simulink model "OneLeg_VR_TouchInput"  (Simulink 7.3)
settings: Solver=ode15s  StartTime=0.0  StopTime=inf  RelTol=1e-3
PreLoadFcn:
  | init_hopper
PostLoadFcn:
  | vrmfunc('FnOpen', [bdroot, '/Data Display and Analysis/VR Sink']);
undefined symbols (not defined in the file or in its folder): body, ctrl, ground, leg, sfuntraj, sigbuilder_block, Traj
libraries: mblibv1 x27, dspmtrx3 x8, simulink x4, vrlib x1
(part 2 of 2)

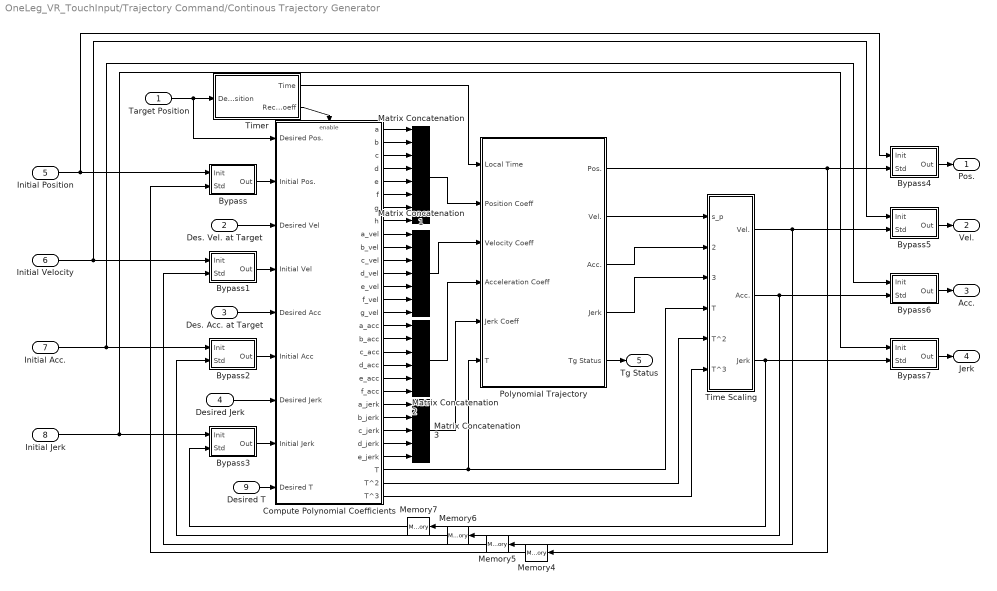
== system OneLeg_VR_TouchInput/Trajectory Command/Continous Trajectory Generator ==
  Target Position : Inport  OutDataType=sfix(16)  OutScaling=2^0
  Des. Vel. at Target : Inport  Port=2  OutDataType=sfix(16)  OutScaling=2^0
  Des. Acc. at Target : Inport  Port=3  OutDataType=sfix(16)  OutScaling=2^0
  Desired Jerk : Inport  Port=4  OutDataType=sfix(16)  OutScaling=2^0
  Initial Position : Inport  Port=5  OutDataType=sfix(16)  OutScaling=2^0
  Initial Velocity : Inport  Port=6  OutDataType=sfix(16)  OutScaling=2^0
  Initial Acc. : Inport  Port=7  OutDataType=sfix(16)  OutScaling=2^0
  Initial Jerk : Inport  Port=8  OutDataType=sfix(16)  OutScaling=2^0
  Desired T : Inport  Port=9  OutDataType=sfix(16)  OutScaling=2^0
  Bypass : Subsystem
  Bypass1 : Subsystem
  Bypass2 : Subsystem
  Bypass3 : Subsystem
  Bypass4 : Subsystem
  Bypass5 : Subsystem
  Bypass6 : Subsystem
  Bypass7 : Subsystem
  Compute Polynomial Coefficients : Subsystem  TreatAsAtomicUnit=on
  Matrix Concatenation : Concatenate  NumInputs=8  Mode=Multidimensional array
  Matrix Concatenation1 : Concatenate  NumInputs=7  Mode=Multidimensional array
  Matrix Concatenation2 : Concatenate  NumInputs=6  Mode=Multidimensional array
  Matrix Concatenation3 : Concatenate  NumInputs=5  Mode=Multidimensional array
  Memory{4..7} (4 alike) : Memory  InheritSampleTime=on
  Polynomial Trajectory : Subsystem  TreatAsAtomicUnit=on
  Time Scaling : Subsystem
  Timer : Subsystem
  Pos. : Outport
  Vel. : Outport  Port=2
  Acc. : Outport  Port=3
  Jerk : Outport  Port=4
  Tg Status : Outport  Port=5
  wires:
  Bypass7/1(Out) -> Jerk/1
  Bypass6/1(Out) -> Acc./1
  Bypass5/1(Out) -> Vel./1
  Bypass4/1(Out) -> Pos./1
  Memory7/1 -> Bypass3/2(Std)
  Memory6/1 -> Bypass2/2(Std)
  Memory5/1 -> Bypass1/2(Std)
  Memory4/1 -> Bypass/2(Std)
  Initial Jerk/1 -> Bypass7/1(Init), Bypass3/1(Init)
  Initial Acc./1 -> Bypass6/1(Init), Bypass2/1(Init)
  Initial Velocity/1 -> Bypass5/1(Init), Bypass1/1(Init)
  Bypass/1(Out) -> Compute Polynomial Coefficients/2(Initial Pos.)
  Initial Position/1 -> Bypass4/1(Init), Bypass/1(Init)
  Compute Polynomial Coefficients/29(T^3) -> Time Scaling/6(T^3)
  Compute Polynomial Coefficients/28(T^2) -> Time Scaling/5(T^2)
  Time Scaling/3(Jerk) -> Bypass7/2(Std), Memory7/1
  Polynomial Trajectory/4(Jerk) -> Time Scaling/3(s_ppp)
  Matrix Concatenation3/1 -> Polynomial Trajectory/5(Jerk Coeff)
  Matrix Concatenation2/1 -> Polynomial Trajectory/4(Acceleration Coeff)
  Matrix Concatenation1/1 -> Polynomial Trajectory/3(Velocity Coeff)
  Matrix Concatenation/1 -> Polynomial Trajectory/2(Position Coeff)
  Compute Polynomial Coefficients/26(e_jerk) -> Matrix Concatenation3/5
  Compute Polynomial Coefficients/25(d_jerk) -> Matrix Concatenation3/4
  Compute Polynomial Coefficients/24(c_jerk) -> Matrix Concatenation3/3
  Compute Polynomial Coefficients/23(b_jerk) -> Matrix Concatenation3/2
  Compute Polynomial Coefficients/22(a_jerk) -> Matrix Concatenation3/1
  Compute Polynomial Coefficients/21(f_acc) -> Matrix Concatenation2/6
  Compute Polynomial Coefficients/20(e_acc) -> Matrix Concatenation2/5
  Compute Polynomial Coefficients/19(d_acc) -> Matrix Concatenation2/4
  Compute Polynomial Coefficients/18(c_acc) -> Matrix Concatenation2/3
  Compute Polynomial Coefficients/17(b_acc) -> Matrix Concatenation2/2
  Compute Polynomial Coefficients/16(a_acc) -> Matrix Concatenation2/1
  Compute Polynomial Coefficients/15(g_vel) -> Matrix Concatenation1/7
  Compute Polynomial Coefficients/14(f_vel) -> Matrix Concatenation1/6
  Compute Polynomial Coefficients/13(e_vel) -> Matrix Concatenation1/5
  Compute Polynomial Coefficients/12(d_vel) -> Matrix Concatenation1/4
  Compute Polynomial Coefficients/11(c_vel) -> Matrix Concatenation1/3
  Compute Polynomial Coefficients/10(b_vel) -> Matrix Concatenation1/2
  Compute Polynomial Coefficients/9(a_vel) -> Matrix Concatenation1/1
  Compute Polynomial Coefficients/8(h) -> Matrix Concatenation/8
  Compute Polynomial Coefficients/7(g) -> Matrix Concatenation/7
  Compute Polynomial Coefficients/6(f) -> Matrix Concatenation/6
  Compute Polynomial Coefficients/5(e) -> Matrix Concatenation/5
  Compute Polynomial Coefficients/4(d) -> Matrix Concatenation/4
  Compute Polynomial Coefficients/3(c) -> Matrix Concatenation/3
  Compute Polynomial Coefficients/2(b) -> Matrix Concatenation/2
  Compute Polynomial Coefficients/1(a) -> Matrix Concatenation/1
  Desired Jerk/1 -> Compute Polynomial Coefficients/7(Desired Jerk)
  Bypass3/1(Out) -> Compute Polynomial Coefficients/8(Initial Jerk)
  Time Scaling/1(Vel.) -> Memory5/1, Bypass5/2(Std)
  Desired T/1 -> Compute Polynomial Coefficients/9(Desired T)
  Time Scaling/2(Acc.) -> Bypass6/2(Std), Memory6/1
  Bypass2/1(Out) -> Compute Polynomial Coefficients/6(Initial Acc)
  Bypass1/1(Out) -> Compute Polynomial Coefficients/4(Initial Vel)
  Timer/2(Recompute Coeff) -> Compute Polynomial Coefficients/Enable
  Des. Acc. at Target/1 -> Compute Polynomial Coefficients/5(Desired Acc)
  Des. Vel. at Target/1 -> Compute Polynomial Coefficients/3(Desired Vel)
  Compute Polynomial Coefficients/27(T) -> Time Scaling/4(T), Polynomial Trajectory/6(T)
  Polynomial Trajectory/5(Tg Status) -> Tg Status/1
  Target Position/1 -> Compute Polynomial Coefficients/1(Desired Pos.), Timer/1(Desired Position)
  Polynomial Trajectory/1(Pos.) -> Bypass4/2(Std), Memory4/1
  Timer/1(Time) -> Polynomial Trajectory/1(Local Time)
  Polynomial Trajectory/3(Acc.) -> Time Scaling/2(s_pp)
  Polynomial Trajectory/2(Vel.) -> Time Scaling/1(s_p)

== system OneLeg_VR_TouchInput/Trajectory Command/Signal Builder ==
  Demux : Demux  Tag=STV Demux  Outputs=1
  FromWs : FromWorkspace  Tag=STV FromWs  VariableName=tuvar  SampleTime=0  SigBuilderData=DataTag1  VnvData=DataTag2
      SigBuilderData=|
      | common.afterFinalStr = 'Extrapolate'
      | common.sampleTime = 0
      | dataSet.timeRange = [0 35]
      | dataSet.name = 'Group 1'
      | sbobj.Groups{1}.Signals{1}.XData = [0 2 8 15 20 35]
      | sbobj.Groups{1}.Signals{1}.YData = [0 0 0.2 0.2 0 0]
  Signal 2 : Outport  Tag=STV Outport
  wires:
  FromWs/1 -> Demux/1
  Demux/1 -> Signal 2/1

== system OneLeg_VR_TouchInput/Trajectory Command/Signal Builder1 ==
  Demux : Demux  Tag=STV Demux  Outputs=1
  FromWs : FromWorkspace  Tag=STV FromWs  VariableName=tuvar  SampleTime=0  SigBuilderData=DataTag3  VnvData=DataTag4
      SigBuilderData=|
      | common.afterFinalStr = 'Extrapolate'
      | common.sampleTime = 0
      | dataSet.timeRange = [0 35]
      | dataSet.name = 'Group 1'
      | sbobj.Groups{1}.Signals{1}.XData = [0 8 12 20 25 35]
      | sbobj.Groups{1}.Signals{1}.YData = [0 0 0.2 0.201 0 0]
  Signal 2 : Outport  Tag=STV Outport
  wires:
  Demux/1 -> Signal 2/1
  FromWs/1 -> Demux/1

== system OneLeg_VR_TouchInput/Trajectory Command/padding ==
  In1 : Inport
  Constant3 : Constant  Value=0  OutDataType=sfix(16)  OutScaling=2^0
  Mux4 : Mux  Inputs=2
  Out1 : Outport
  wires:
  Constant3/1 -> Mux4/2
  Mux4/1 -> Out1/1
  In1/1 -> Mux4/1

== system OneLeg_VR_TouchInput/Control/Motion analysis/Compute Jump Duration ==
  Enable : EnablePort  StatesWhenEnabling=reset
  Integrator1 : Integrator
  X torque2 : Constant  OutDataType=sfix(16)  OutScaling=2^0
  t : Outport  InitialOutput=[.45]
  wires:
  X torque2/1 -> Integrator1/1
  Integrator1/1 -> t/1

== system OneLeg_VR_TouchInput/Control/Motion analysis/Compute Stance Duration ==
  Enable : EnablePort  StatesWhenEnabling=reset
  Integrator1 : Integrator
  X torque2 : Constant  OutDataType=sfix(16)  OutScaling=2^0
  t : Outport  InitialOutput=[.16]
  wires:
  X torque2/1 -> Integrator1/1
  Integrator1/1 -> t/1

== system OneLeg_VR_TouchInput/Control/Motion analysis/Keep First ==
  x : Inport  OutDataType=sfix(16)  OutScaling=2^0
  Trigger : TriggerPort
  x0 : Outport  OutDataType=sfix(16)  OutScaling=2^0
  wires:
  x/1 -> x0/1

== system OneLeg_VR_TouchInput/Control/Motion analysis/Store Jump Duration ==
  T up : Inport  OutDataType=sfix(16)  OutScaling=2^0
  Trigger : TriggerPort  TriggerType=falling
  T up k : Outport  OutDataType=sfix(16)  OutScaling=2^0  InitialOutput=[.45]
  wires:
  T up/1 -> T up k/1  "Jump Duration"

== system OneLeg_VR_TouchInput/Control/Motion analysis/Store Stance Duration ==
  t stance : Inport  OutDataType=sfix(16)  OutScaling=2^0
  x0 : Inport  Port=2  OutDataType=sfix(16)  OutScaling=2^0
  x : Inport  Port=3  OutDataType=sfix(16)  OutScaling=2^0
  Trigger : TriggerPort  TriggerType=falling
  Divide : Product  Inputs=*/  OutDataType=sfix(16)  OutScaling=2^-10
  Sum : Sum  Inputs=+-  OutDataType=sfix(16)  OutScaling=2^0
  V avg : Outport  OutDataType=sfix(16)  OutScaling=2^0
  X stance : Outport  Port=2  OutDataType=sfix(16)  OutScaling=2^0
  wires:
  x/1 -> Sum/2
  x0/1 -> Sum/1
  Sum/1 -> X stance/1, Divide/1
  t stance/1 -> Divide/2  "Stance Duration"
  Divide/1 -> V avg/1

== system OneLeg_VR_TouchInput/Control/Velocity Control/Linear TrajGen ==
  Duration : Inport
  xd : Inport  Port=2
  x0 : Inport  Port=3
  Detect Change : Subsystem
  Enabled Subsystem : Subsystem  TreatAsAtomicUnit=on
  Integrator : Integrator  ExternalReset=rising
  Output Of Traj Gen : Sum  OutDataType=sfix(16)  OutScaling=2^-10
  Product : Product  Inputs=/*  OutDataType=sfix(16)  OutScaling=2^0  RndMeth=Zero
  Product1 : Product  Inputs=**  OutDataType=sfix(16)  OutScaling=2^0  RndMeth=Zero
  Saturation Dynamic : simulink/Discontinuities/Saturation Dynamic  SystemSampleTime=-1  OutMin=[]  OutMax=[]  OutDataTypeStr=Inherit: Same as second input  OutDataType=sfix(16)  OutScaling=2^-10  DoSatur=off
  Subtract : Sum  Inputs=+-  OutDataType=sfix(16)  OutScaling=2^-10
  one : Constant  OutDataType=sfix(16)  OutScaling=2^0
  one1 : Constant  Value=0  OutDataType=sfix(16)  OutScaling=2^0
  x : Outport
  wires:
  x0/1 -> Enabled Subsystem/1(In1)
  Output Of Traj Gen/1 -> x/1
  Detect Change/1(Y) -> Integrator/2, Enabled Subsystem/Enable
  Product1/1 -> Output Of Traj Gen/1
  Product/1 -> Product1/1  "Time"
  one1/1 -> Saturation Dynamic/3
  Duration/1 -> Saturation Dynamic/1, Product/1
  Saturation Dynamic/1 -> Product/2
  Subtract/1 -> Product1/2  "Distance"
  Integrator/1 -> Saturation Dynamic/2
  one/1 -> Integrator/1
  Enabled Subsystem/1(Out1) -> Output Of Traj Gen/2, Subtract/2  "Initial Position"
  xd/1 -> Detect Change/1(U), Subtract/1

== system OneLeg_VR_TouchInput/Robot/Leg Tip and Contact Dynamics/Contact Force ==
  Body Actuator : mblibv1/Sensors &  Actuators/Body Actuator  DialogController=MECH.DynMechDlgSource  SystemSampleTime=-1  UpdateFromCAD=off  PhysicalDomain=Mechanical  PortType=blob  ActuationStyle=Force  AngleUnits=deg  ArcVelocityUnits=deg/s  ArcAccelerationUnits=deg/s^2  CoordPositionUnits=m  VelocityUnits=m/s  AccelerationUnits=m/s^2  ForceUnits=N  TorqueUnits=N*m  ActiveIO=on  Width=3  DialogClass=MechanicalActuatorBlock  ReferenceFrame=Absolute (World)  Angle=off  CoordPosition=on  Force=on  Torque=off
  Body Sensor : mblibv1/Sensors &  Actuators/Body Sensor  DialogController=MECH.DynMechDlgSource  SystemSampleTime=-1  UpdateFromCAD=off  PhysicalDomain=Mechanical  PortType=blob  Muxed=off  Pose=off  Angle=on  AngleUnits=deg  ArcVelocity=off  ArcVelocityUnits=deg/s  ArcAcceleration=off  ArcAccelerationUnits=deg/s^2  CoordPosition=on  CoordPositionUnits=m  Velocity=on  VelocityUnits=m/s  Acceleration=off  AccelerationUnits=m/s^2  Quaternion=on  QuaternionDT=off  QuaternionDDT=off  QuaternionUnits=off  OutputVector=[ 3 3 ]  ActiveIO=on  Width=6  DialogClass=MechanicalSensorBlock  ReferenceFrame=Absolute (World)
  Force Law : Subsystem
  Mechanical Branching Bar : mblibv1/Utilities/Mechanical Branching Bar  DialogController=MECH.DynMechDlgSource  PhysicalDomain=mechanical  SubClassName=Unknown  LeftPortType=blob  RightPortType=blob  LConnTagsString=_newl0  RConnTagsString=__newr0|SA2  UpdateFromCAD=off  DialogClass=MechanicalBranchingBarBlock  NumSAPorts=2
  Tip : PMIOPort  Tag=PMCPort  Port=1  Side=Right
  Position : Outport  OutDataType=sfix(16)  OutScaling=2^0
  Contact Force : Outport  Port=2  OutDataType=sfix(16)  OutScaling=2^0
  wires:
  Body Sensor/1 -> Position/1, Force Law/1(pos)  "Position (m)"
  Body Sensor/2 -> Force Law/2(vel)  "Velocity (m/s)"
  Force Law/1(force) -> Body Actuator/1, Contact Force/1  "Force (N)"
  connections:
  Mechanical Branching Bar/LConn1 -- Tip/RConn1
  Body Actuator/RConn1 -- Mechanical Branching Bar/RConn2
  Body Sensor/LConn1 -- Mechanical Branching Bar/RConn1

== system OneLeg_VR_TouchInput/Trajectory Command/Continous Trajectory Generator/Bypass ==
  Init : Inport  OutDataType=sfix(16)  OutScaling=2^0
  Std : Inport  Port=2  OutDataType=sfix(16)  OutScaling=2^0
  Constant : Constant  Value=0  OutDataType=sfix(16)  OutScaling=2^0  SampleTime=st
  Memory : Memory  X0=1  InheritSampleTime=on
  Signal Specification : SignalSpecification  SampleTime=st  OutDataType=sfix(16)  OutScaling=2^0
  Switch3 : Switch  Threshold=0.5  SaturateOnIntegerOverflow=on
  Out : Outport
  wires:
  Memory/1 -> Switch3/2
  Std/1 -> Switch3/3
  Switch3/1 -> Signal Specification/1
  Init/1 -> Switch3/1
  Constant/1 -> Memory/1
  Signal Specification/1 -> Out/1

== system OneLeg_VR_TouchInput/Trajectory Command/Continous Trajectory Generator/Bypass1 ==
  Init : Inport  OutDataType=sfix(16)  OutScaling=2^0
  Std : Inport  Port=2  OutDataType=sfix(16)  OutScaling=2^0
  Constant : Constant  Value=0  OutDataType=sfix(16)  OutScaling=2^0  SampleTime=st
  Memory : Memory  X0=1  InheritSampleTime=on
  Signal Specification : SignalSpecification  SampleTime=st  OutDataType=sfix(16)  OutScaling=2^0
  Switch3 : Switch  Threshold=0.5  SaturateOnIntegerOverflow=on
  Out : Outport
  wires:
  Memory/1 -> Switch3/2
  Constant/1 -> Memory/1
  Init/1 -> Switch3/1
  Switch3/1 -> Signal Specification/1
  Std/1 -> Switch3/3
  Signal Specification/1 -> Out/1

== system OneLeg_VR_TouchInput/Trajectory Command/Continous Trajectory Generator/Bypass2 ==
  Init : Inport  OutDataType=sfix(16)  OutScaling=2^0
  Std : Inport  Port=2  OutDataType=sfix(16)  OutScaling=2^0
  Constant : Constant  Value=0  OutDataType=sfix(16)  OutScaling=2^0  SampleTime=st
  Memory : Memory  X0=1  InheritSampleTime=on
  Signal Specification : SignalSpecification  SampleTime=st  OutDataType=sfix(16)  OutScaling=2^0
  Switch3 : Switch  Threshold=0.5  SaturateOnIntegerOverflow=on
  Out : Outport
  wires:
  Memory/1 -> Switch3/2
  Constant/1 -> Memory/1
  Std/1 -> Switch3/3
  Switch3/1 -> Signal Specification/1
  Init/1 -> Switch3/1
  Signal Specification/1 -> Out/1

== system OneLeg_VR_TouchInput/Trajectory Command/Continous Trajectory Generator/Bypass3 ==
  Init : Inport  OutDataType=sfix(16)  OutScaling=2^0
  Std : Inport  Port=2  OutDataType=sfix(16)  OutScaling=2^0
  Constant1 : Constant  Value=0  OutDataType=sfix(16)  OutScaling=2^0  SampleTime=st
  Memory : Memory  X0=1  InheritSampleTime=on
  Signal Specification : SignalSpecification  SampleTime=st  OutDataType=sfix(16)  OutScaling=2^0
  Switch3 : Switch  Threshold=0.5  SaturateOnIntegerOverflow=on
  Out : Outport
  wires:
  Constant1/1 -> Memory/1
  Init/1 -> Switch3/1
  Switch3/1 -> Signal Specification/1
  Std/1 -> Switch3/3
  Memory/1 -> Switch3/2
  Signal Specification/1 -> Out/1

== system OneLeg_VR_TouchInput/Trajectory Command/Continous Trajectory Generator/Bypass4 ==
  Init : Inport  OutDataType=sfix(16)  OutScaling=2^0
  Std : Inport  Port=2  OutDataType=sfix(16)  OutScaling=2^0
  Constant1 : Constant  Value=0  OutDataType=sfix(16)  OutScaling=2^0  SampleTime=st
  Memory : Memory  X0=1  InheritSampleTime=on
  Switch3 : Switch  Threshold=0.5  SaturateOnIntegerOverflow=on
  Out : Outport
  wires:
  Constant1/1 -> Memory/1
  Init/1 -> Switch3/1
  Switch3/1 -> Out/1
  Std/1 -> Switch3/3
  Memory/1 -> Switch3/2

== system OneLeg_VR_TouchInput/Trajectory Command/Continous Trajectory Generator/Bypass5 ==
  Init : Inport  OutDataType=sfix(16)  OutScaling=2^0
  Std : Inport  Port=2  OutDataType=sfix(16)  OutScaling=2^0
  Constant1 : Constant  Value=0  OutDataType=sfix(16)  OutScaling=2^0  SampleTime=st
  Memory : Memory  X0=1  InheritSampleTime=on
  Switch3 : Switch  Threshold=0.5  SaturateOnIntegerOverflow=on
  Out : Outport
  wires:
  Memory/1 -> Switch3/2
  Std/1 -> Switch3/3
  Switch3/1 -> Out/1
  Init/1 -> Switch3/1
  Constant1/1 -> Memory/1

== system OneLeg_VR_TouchInput/Trajectory Command/Continous Trajectory Generator/Bypass6 ==
  Init : Inport  OutDataType=sfix(16)  OutScaling=2^0
  Std : Inport  Port=2  OutDataType=sfix(16)  OutScaling=2^0
  Constant1 : Constant  Value=0  OutDataType=sfix(16)  OutScaling=2^0  SampleTime=st
  Memory : Memory  X0=1  InheritSampleTime=on
  Switch3 : Switch  Threshold=0.5  SaturateOnIntegerOverflow=on
  Out : Outport
  wires:
  Constant1/1 -> Memory/1
  Init/1 -> Switch3/1
  Switch3/1 -> Out/1
  Std/1 -> Switch3/3
  Memory/1 -> Switch3/2

== system OneLeg_VR_TouchInput/Trajectory Command/Continous Trajectory Generator/Bypass7 ==
  Init : Inport  OutDataType=sfix(16)  OutScaling=2^0
  Std : Inport  Port=2  OutDataType=sfix(16)  OutScaling=2^0
  Constant1 : Constant  Value=0  OutDataType=sfix(16)  OutScaling=2^0  SampleTime=st
  Memory : Memory  X0=1  InheritSampleTime=on
  Switch3 : Switch  Threshold=0.5  SaturateOnIntegerOverflow=on
  Out : Outport
  wires:
  Memory/1 -> Switch3/2
  Std/1 -> Switch3/3
  Switch3/1 -> Out/1
  Init/1 -> Switch3/1
  Constant1/1 -> Memory/1

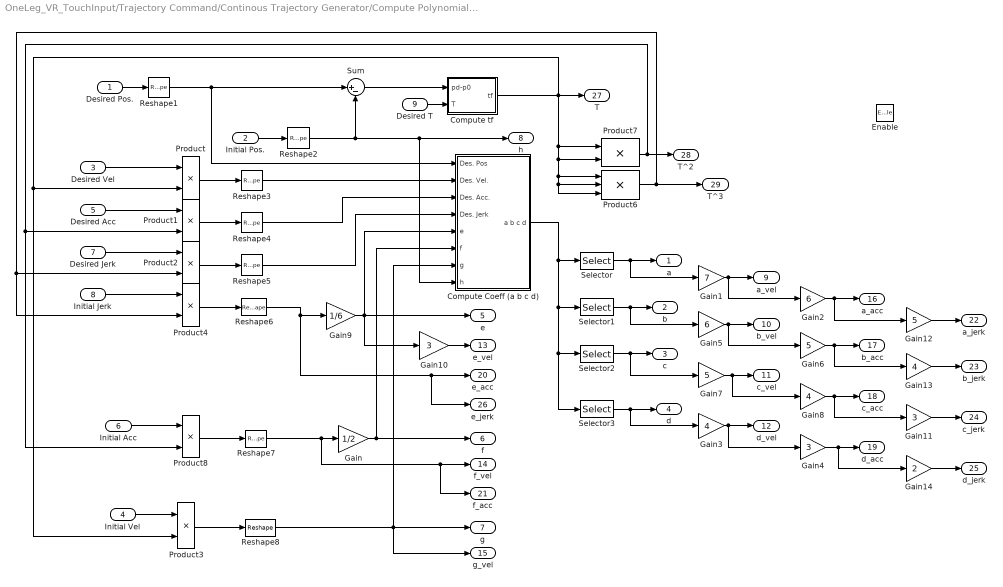
== system OneLeg_VR_TouchInput/Trajectory Command/Continous Trajectory Generator/Compute Polynomial Coefficients ==
  Desired Pos. : Inport  OutDataType=sfix(16)  OutScaling=2^0
  Initial Pos. : Inport  Port=2  OutDataType=sfix(16)  OutScaling=2^0
  Desired Vel : Inport  Port=3  OutDataType=sfix(16)  OutScaling=2^0
  Initial Vel : Inport  Port=4  OutDataType=sfix(16)  OutScaling=2^0
  Desired Acc : Inport  Port=5  OutDataType=sfix(16)  OutScaling=2^0
  Initial Acc : Inport  Port=6  OutDataType=sfix(16)  OutScaling=2^0
  Desired Jerk : Inport  Port=7  OutDataType=sfix(16)  OutScaling=2^0
  Initial Jerk : Inport  Port=8  OutDataType=sfix(16)  OutScaling=2^0
  Desired T : Inport  Port=9  OutDataType=sfix(16)  OutScaling=2^0
  Enable : EnablePort  StatesWhenEnabling=reset
  Compute Coeff (a b c d) : Subsystem
  Compute tf : Subsystem
  Gain : Gain  Gain=1/2  ParameterDataType=sfix(16)  ParameterScaling=2^0  OutDataType=sfix(16)  OutScaling=2^0  SaturateOnIntegerOverflow=on  OutDataTypeStr=Inherit: Same as input  ParamDataTypeStr=Inherit: Same as input
  Gain1 : Gain  Gain=7  ParameterDataType=sfix(16)  ParameterScaling=2^0  OutDataType=sfix(16)  OutScaling=2^0  SaturateOnIntegerOverflow=on  OutDataTypeStr=Inherit: Same as input  ParamDataTypeStr=Inherit: Same as input
  Gain10 : Gain  Gain=3  ParameterDataType=sfix(16)  ParameterScaling=2^0  OutDataType=sfix(16)  OutScaling=2^0  SaturateOnIntegerOverflow=on  OutDataTypeStr=Inherit: Same as input  ParamDataTypeStr=Inherit: Same as input
  Gain11 : Gain  Gain=3  ParameterDataType=sfix(16)  ParameterScaling=2^0  OutDataType=sfix(16)  OutScaling=2^0  SaturateOnIntegerOverflow=on  OutDataTypeStr=Inherit: Same as input  ParamDataTypeStr=Inherit: Same as input
  Gain12 : Gain  Gain=5  ParameterDataType=sfix(16)  ParameterScaling=2^0  OutDataType=sfix(16)  OutScaling=2^0  SaturateOnIntegerOverflow=on  OutDataTypeStr=Inherit: Same as input  ParamDataTypeStr=Inherit: Same as input
  Gain13 : Gain  Gain=4  ParameterDataType=sfix(16)  ParameterScaling=2^0  OutDataType=sfix(16)  OutScaling=2^0  SaturateOnIntegerOverflow=on  OutDataTypeStr=Inherit: Same as input  ParamDataTypeStr=Inherit: Same as input
  Gain14 : Gain  Gain=2  ParameterDataType=sfix(16)  ParameterScaling=2^0  OutDataType=sfix(16)  OutScaling=2^0  SaturateOnIntegerOverflow=on  OutDataTypeStr=Inherit: Same as input  ParamDataTypeStr=Inherit: Same as input
  Gain2 : Gain  Gain=6  ParameterDataType=sfix(16)  ParameterScaling=2^0  OutDataType=sfix(16)  OutScaling=2^0  SaturateOnIntegerOverflow=on  OutDataTypeStr=Inherit: Same as input  ParamDataTypeStr=Inherit: Same as input
  Gain3 : Gain  Gain=4  ParameterDataType=sfix(16)  ParameterScaling=2^0  OutDataType=sfix(16)  OutScaling=2^0  SaturateOnIntegerOverflow=on  OutDataTypeStr=Inherit: Same as input  ParamDataTypeStr=Inherit: Same as input
  Gain4 : Gain  Gain=3  ParameterDataType=sfix(16)  ParameterScaling=2^0  OutDataType=sfix(16)  OutScaling=2^0  SaturateOnIntegerOverflow=on  OutDataTypeStr=Inherit: Same as input  ParamDataTypeStr=Inherit: Same as input
  Gain5 : Gain  Gain=6  ParameterDataType=sfix(16)  ParameterScaling=2^0  OutDataType=sfix(16)  OutScaling=2^0  SaturateOnIntegerOverflow=on  OutDataTypeStr=Inherit: Same as input  ParamDataTypeStr=Inherit: Same as input
  Gain6 : Gain  Gain=5  ParameterDataType=sfix(16)  ParameterScaling=2^0  OutDataType=sfix(16)  OutScaling=2^0  SaturateOnIntegerOverflow=on  OutDataTypeStr=Inherit: Same as input  ParamDataTypeStr=Inherit: Same as input
  Gain7 : Gain  Gain=5  ParameterDataType=sfix(16)  ParameterScaling=2^0  OutDataType=sfix(16)  OutScaling=2^0  SaturateOnIntegerOverflow=on  OutDataTypeStr=Inherit: Same as input  ParamDataTypeStr=Inherit: Same as input
  Gain8 : Gain  Gain=4  ParameterDataType=sfix(16)  ParameterScaling=2^0  OutDataType=sfix(16)  OutScaling=2^0  SaturateOnIntegerOverflow=on  OutDataTypeStr=Inherit: Same as input  ParamDataTypeStr=Inherit: Same as input
  Gain9 : Gain  Gain=1/6  ParameterDataType=sfix(16)  ParameterScaling=2^0  OutDataType=sfix(16)  OutScaling=2^0  SaturateOnIntegerOverflow=on  OutDataTypeStr=Inherit: Same as input  ParamDataTypeStr=Inherit: Same as input
  Product{,1..4,7..8} (7 alike) : Product  OutDataType=sfix(16)  OutScaling=2^0  SaturateOnIntegerOverflow=on  OutDataTypeStr=Inherit: Same as first input
  Product6 : Product  Inputs=3  OutDataType=sfix(16)  OutScaling=2^0  SaturateOnIntegerOverflow=on  OutDataTypeStr=Inherit: Same as first input
  Reshape{1..8} (8 alike) : Reshape  OutputDimensionality=Row vector (2-D)
  Selector : Selector  NumberOfDimensions=2  InputPortWidth=3  IndexOptions=Index vector (dialog),Select all  Indices=1,-1  OutputSizes=1
  Selector1 : Selector  NumberOfDimensions=2  InputPortWidth=3  IndexOptions=Index vector (dialog),Select all  Indices=2,-1  OutputSizes=1
  Selector2 : Selector  NumberOfDimensions=2  InputPortWidth=3  IndexOptions=Index vector (dialog),Select all  Indices=3,-1  OutputSizes=1
  Selector3 : Selector  NumberOfDimensions=2  InputPortWidth=3  IndexOptions=Index vector (dialog),Select all  Indices=4,-1  OutputSizes=1
  Sum : Sum  Inputs=|+-  OutDataType=sfix(16)  OutScaling=2^0  SaturateOnIntegerOverflow=on  InputSameDT=on  OutDataTypeStr=Inherit: Same as first input
  a : Outport
  b : Outport  Port=2
  c : Outport  Port=3
  d : Outport  Port=4
  e : Outport  Port=5
  f : Outport  Port=6
  g : Outport  Port=7
  h : Outport  Port=8
  a_vel : Outport  Port=9
  b_vel : Outport  Port=10
  c_vel : Outport  Port=11
  d_vel : Outport  Port=12
  e_vel : Outport  Port=13
  f_vel : Outport  Port=14
  g_vel : Outport  Port=15
  a_acc : Outport  Port=16
  b_acc : Outport  Port=17
  c_acc : Outport  Port=18
  d_acc : Outport  Port=19
  e_acc : Outport  Port=20
  f_acc : Outport  Port=21
  a_jerk : Outport  Port=22
  b_jerk : Outport  Port=23
  c_jerk : Outport  Port=24
  d_jerk : Outport  Port=25
  e_jerk : Outport  Port=26
  T : Outport  Port=27
  T^2 : Outport  Port=28
  T^3 : Outport  Port=29
  wires:
  Product6/1 -> Product4/2, Product2/2, T^3/1
  Product7/1 -> Product1/2, Product8/2, T^2/1
  Product1/1 -> Reshape4/1
  Desired Acc/1 -> Product1/1
  Product2/1 -> Reshape5/1
  Desired Jerk/1 -> Product2/1
  Product4/1 -> Reshape6/1
  Initial Jerk/1 -> Product4/1
  Product8/1 -> Reshape7/1
  Product3/1 -> Reshape8/1
  Product/1 -> Reshape3/1
  Desired Vel/1 -> Product/1
  Reshape8/1 -> Compute Coeff (a b c d)/7(g), g/1, g_vel/1
  Reshape7/1 -> f_acc/1, f_vel/1, Gain/1
  Reshape6/1 -> e_jerk/1, e_acc/1, Gain9/1
  Reshape5/1 -> Compute Coeff (a b c d)/4(Des. Jerk)
  Reshape4/1 -> Compute Coeff (a b c d)/3(Des. Acc.)
  Reshape3/1 -> Compute Coeff (a b c d)/2(Des. Vel.)
  Reshape2/1 -> Compute Coeff (a b c d)/8(h), h/1, Sum/2
  Reshape1/1 -> Compute Coeff (a b c d)/1(Des. Pos), Sum/1
  Gain14/1 -> d_jerk/1
  Gain11/1 -> c_jerk/1
  Gain13/1 -> b_jerk/1
  Gain12/1 -> a_jerk/1
  Gain10/1 -> e_vel/1
  Gain9/1 -> e/1, Compute Coeff (a b c d)/5(e), Gain10/1
  Gain4/1 -> Gain14/1, d_acc/1
  Gain3/1 -> d_vel/1, Gain4/1
  Selector3/1 -> Gain3/1, d/1
  Desired T/1 -> Compute tf/2(T)
  Gain/1 -> Compute Coeff (a b c d)/6(f), f/1
  Gain8/1 -> Gain11/1, c_acc/1
  Gain7/1 -> Gain8/1, c_vel/1
  Gain6/1 -> Gain13/1, b_acc/1
  Gain5/1 -> Gain6/1, b_vel/1
  Gain2/1 -> Gain12/1, a_acc/1
  Gain1/1 -> Gain2/1, a_vel/1
  Compute tf/1(tf) -> Product6/3, Product6/2, Product6/1, Product7/2, Product7/1, T/1, Product3/2, Product/2
  Initial Vel/1 -> Product3/1
  Initial Acc/1 -> Product8/1
  Selector2/1 -> Gain7/1, c/1
  Selector1/1 -> Gain5/1, b/1
  Selector/1 -> a/1, Gain1/1
  Compute Coeff (a b c d)/1(a b c d) -> Selector3/1, Selector2/1, Selector/1, Selector1/1
  Sum/1 -> Compute tf/1(pd-p0)
  Initial Pos./1 -> Reshape2/1
  Desired Pos./1 -> Reshape1/1

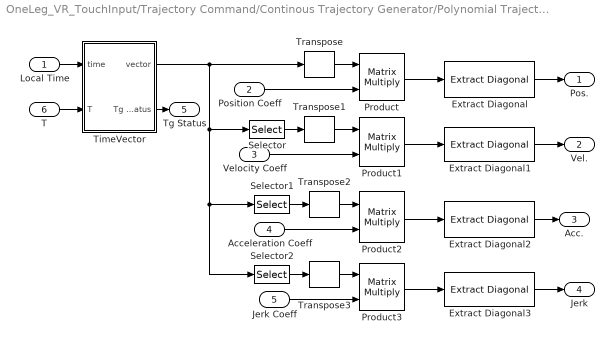
== system OneLeg_VR_TouchInput/Trajectory Command/Continous Trajectory Generator/Polynomial Trajectory ==
  Local Time : Inport  OutDataType=sfix(16)  OutScaling=2^0
  Position Coeff : Inport  Port=2  OutDataType=sfix(16)  OutScaling=2^0
  Velocity Coeff : Inport  Port=3  OutDataType=sfix(16)  OutScaling=2^0
  Acceleration Coeff : Inport  Port=4  OutDataType=sfix(16)  OutScaling=2^0
  Jerk Coeff : Inport  Port=5  OutDataType=sfix(16)  OutScaling=2^0
  T : Inport  Port=6  OutDataType=sfix(16)  OutScaling=2^0
  Extract Diagonal{,1..3} (4 alike) : dspmtrx3/Extract Diagonal
  Product{,1..3} (4 alike) : Product  Multiplication=Matrix(*)  OutDataType=sfix(16)  OutScaling=2^0  SaturateOnIntegerOverflow=on  OutDataTypeStr=Inherit: Same as first input
  Selector : Selector  NumberOfDimensions=2  InputPortWidth=7  IndexOptions=Index vector (dialog),Select all  Indices=[ 2 3 4 5 6 7 8],-1  OutputSizes=1
  Selector1 : Selector  NumberOfDimensions=2  InputPortWidth=7  IndexOptions=Index vector (dialog),Select all  Indices="[  3 4 5 6 7 8],-1"  OutputSizes=1
  Selector2 : Selector  NumberOfDimensions=2  InputPortWidth=7  IndexOptions=Index vector (dialog),Select all  Indices="[   4 5 6 7 8],-1"  OutputSizes=1
  TimeVector : Subsystem
  Transpose{,1..3} (4 alike) : dspmtrx3/Transpose  SystemSampleTime=-1  Hermitian=off  overflowFlag=off
  Pos. : Outport
  Vel. : Outport  Port=2
  Acc. : Outport  Port=3
  Jerk : Outport  Port=4
  Tg Status : Outport  Port=5
  wires:
  Extract Diagonal3/1 -> Jerk/1
  Extract Diagonal2/1 -> Acc./1
  Extract Diagonal1/1 -> Vel./1
  Extract Diagonal/1 -> Pos./1
  Transpose3/1 -> Product3/1
  Transpose2/1 -> Product2/1
  Transpose1/1 -> Product1/1
  Transpose/1 -> Product/1
  Product/1 -> Extract Diagonal/1
  Product2/1 -> Extract Diagonal2/1
  Product1/1 -> Extract Diagonal1/1
  Acceleration Coeff/1 -> Product2/2
  Local Time/1 -> TimeVector/1(time)
  T/1 -> TimeVector/2(T)
  Position Coeff/1 -> Product/2
  Velocity Coeff/1 -> Product1/2
  TimeVector/1(vector) -> Selector/1, Selector2/1, Selector1/1, Transpose/1
  Jerk Coeff/1 -> Product3/2
  Product3/1 -> Extract Diagonal3/1
  Selector/1 -> Transpose1/1
  Selector1/1 -> Transpose2/1
  Selector2/1 -> Transpose3/1
  TimeVector/2(Tg Status) -> Tg Status/1

== system OneLeg_VR_TouchInput/Trajectory Command/Continous Trajectory Generator/Time Scaling ==
  s_p : Inport  OutDataType=sfix(16)  OutScaling=2^0
  s_pp : Inport  Port=2  OutDataType=sfix(16)  OutScaling=2^0
  s_ppp : Inport  Port=3  OutDataType=sfix(16)  OutScaling=2^0
  T : Inport  Port=4  OutDataType=sfix(16)  OutScaling=2^0
  T^2 : Inport  Port=5  OutDataType=sfix(16)  OutScaling=2^0
  T^3 : Inport  Port=6  OutDataType=sfix(16)  OutScaling=2^0
  Product1 : Product  Inputs=*/  OutDataType=sfix(16)  OutScaling=2^0  SaturateOnIntegerOverflow=on  OutDataTypeStr=Inherit: Same as first input
  Product2 : Product  Inputs=*/  OutDataType=sfix(16)  OutScaling=2^0  SaturateOnIntegerOverflow=on  OutDataTypeStr=Inherit: Same as first input
  Product3 : Product  Inputs=*/  OutDataType=sfix(16)  OutScaling=2^0  SaturateOnIntegerOverflow=on  OutDataTypeStr=Inherit: Same as first input
  Vel. : Outport
  Acc. : Outport  Port=2
  Jerk : Outport  Port=3
  wires:
  T^2/1 -> Product1/2
  T^3/1 -> Product3/2
  T/1 -> Product2/2
  Product3/1 -> Jerk/1
  s_ppp/1 -> Product3/1
  Product2/1 -> Vel./1
  Product1/1 -> Acc./1
  s_pp/1 -> Product1/1
  s_p/1 -> Product2/1

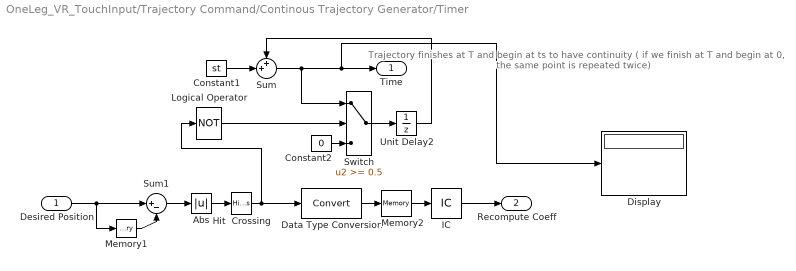
== system OneLeg_VR_TouchInput/Trajectory Command/Continous Trajectory Generator/Timer ==
  note: Trajectory finishes at T and begin at ts
      | to have continuity ( if we finish at T and begin at 0,
      | the same point is repeated twice)
  Desired Position : Inport  OutDataType=sfix(16)  OutScaling=2^0
  Abs : Abs  SaturateOnIntegerOverflow=on
  Constant1 : Constant  Value=st  OutDataType=sfix(16)  OutScaling=2^0  SampleTime=.01
  Constant2 : Constant  Value=0  OutDataType=sfix(16)  OutScaling=2^0
  Data Type Conversion : DataTypeConversion  SaturateOnIntegerOverflow=on  RndMeth=Zero
  Display : Display
  Hit  Crossing : HitCross  HitCrossingOffset=UpdateLimit  HitCrossingDirection=rising
  IC : InitialCondition
  Logical Operator : Logic  Operator=NOT  AllPortsSameDT=off
  Memory1 : Memory  InheritSampleTime=on
  Memory2 : Memory  InheritSampleTime=on
  Sum : Sum  Inputs=++|  OutDataType=sfix(16)  OutScaling=2^0  SaturateOnIntegerOverflow=on  InputSameDT=on  OutDataTypeStr=Inherit: Same as first input
  Sum1 : Sum  Inputs=|+-  OutDataType=sfix(16)  OutScaling=2^0  SaturateOnIntegerOverflow=on
  Switch : Switch  Threshold=0.5  SaturateOnIntegerOverflow=on
  Unit Delay2 : UnitDelay  SampleTime=st
  Time : Outport
  Recompute Coeff : Outport  Port=2
  wires:
  Memory2/1 -> IC/1
  Logical Operator/1 -> Switch/2
  Data Type Conversion/1 -> Memory2/1
  IC/1 -> Recompute Coeff/1
  Abs/1 -> Hit  Crossing/1
  Hit  Crossing/1 -> Data Type Conversion/1, Logical Operator/1
  Memory1/1 -> Sum1/2
  Sum1/1 -> Abs/1
  Switch/1 -> Unit Delay2/1
  Constant2/1 -> Switch/3
  Desired Position/1 -> Sum1/1, Memory1/1
  Unit Delay2/1 -> Sum/1
  Constant1/1 -> Sum/2
  Sum/1 -> Switch/1, Time/1, Display/1

== system OneLeg_VR_TouchInput/Control/Velocity Control/Linear TrajGen/Detect Change ==
  note: U(k)
  note: Edge
  U : Inport  OutDataType=sfix(16)  OutScaling=2^0
  FixPt Relational Operator : RelationalOperator  Operator=~=  LogicOutDataTypeMode=boolean  OutDataTypeStr=boolean  ZeroCross=off
  Memory : Memory
  Y : Outport  OutDataType=sfix(16)  OutScaling=2^0  InitialOutput=0
  wires:
  U/1 -> FixPt Relational Operator/1, Memory/1
  Memory/1 -> FixPt Relational Operator/2  "U(k-1)"
  FixPt Relational Operator/1 -> Y/1

== system OneLeg_VR_TouchInput/Control/Velocity Control/Linear TrajGen/Enabled Subsystem ==
  In1 : Inport  OutDataType=sfix(16)  OutScaling=2^0
  Enable : EnablePort
  Out1 : Outport  OutDataType=sfix(16)  OutScaling=2^0
  wires:
  In1/1 -> Out1/1

== system OneLeg_VR_TouchInput/Robot/Leg Tip and Contact Dynamics/Contact Force/Force Law ==
  pos : Inport  OutDataType=sfix(16)  OutScaling=2^0
  vel : Inport  Port=2  OutDataType=sfix(16)  OutScaling=2^0
  Contact Force : Subsystem  TreatAsAtomicUnit=on
  If : If  IfExpression=u1 < 0
  Merge : Merge  InitialOutput=0  InputPortOffsets=0
  Selector : Selector  InputPortWidth=3  IndexOptions=Index vector (dialog)  Indices=[2]  OutputSizes=1
  Zero Force : Subsystem  TreatAsAtomicUnit=on
  force : Outport  OutDataType=sfix(16)  OutScaling=2^0
  wires:
  Selector/1 -> If/1
  If/1 -> Contact Force/Action
  Merge/1 -> force/1
  Zero Force/1(force) -> Merge/2
  Contact Force/1(force) -> Merge/1
  If/2 -> Zero Force/Action
  vel/1 -> Contact Force/2(vel)
  pos/1 -> Contact Force/1(pos), Selector/1

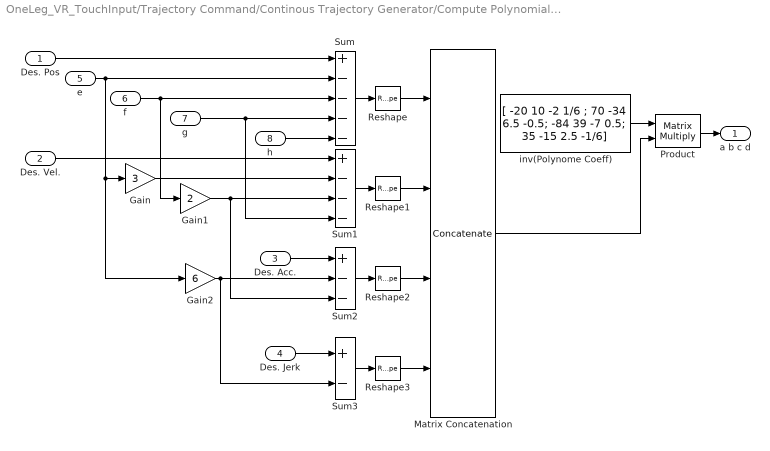
== system OneLeg_VR_TouchInput/Trajectory Command/Continous Trajectory Generator/Compute Polynomial Coefficients/Compute Coeff (a b c d) ==
  Des. Pos : Inport  OutDataType=sfix(16)  OutScaling=2^0
  Des. Vel. : Inport  Port=2  OutDataType=sfix(16)  OutScaling=2^0
  Des. Acc. : Inport  Port=3  OutDataType=sfix(16)  OutScaling=2^0
  Des. Jerk : Inport  Port=4  OutDataType=sfix(16)  OutScaling=2^0
  e : Inport  Port=5  OutDataType=sfix(16)  OutScaling=2^0
  f : Inport  Port=6  OutDataType=sfix(16)  OutScaling=2^0
  g : Inport  Port=7  OutDataType=sfix(16)  OutScaling=2^0
  h : Inport  Port=8  OutDataType=sfix(16)  OutScaling=2^0
  Gain : Gain  Gain=3  ParameterDataType=sfix(16)  ParameterScaling=2^0  OutDataType=sfix(16)  OutScaling=2^0  SaturateOnIntegerOverflow=on  OutDataTypeStr=Inherit: Same as input  ParamDataTypeStr=Inherit: Same as input
  Gain1 : Gain  Gain=2  ParameterDataType=sfix(16)  ParameterScaling=2^0  OutDataType=sfix(16)  OutScaling=2^0  SaturateOnIntegerOverflow=on  OutDataTypeStr=Inherit: Same as input  ParamDataTypeStr=Inherit: Same as input
  Gain2 : Gain  Gain=6  ParameterDataType=sfix(16)  ParameterScaling=2^0  OutDataType=sfix(16)  OutScaling=2^0  SaturateOnIntegerOverflow=on  OutDataTypeStr=Inherit: Same as input  ParamDataTypeStr=Inherit: Same as input
  Matrix Concatenation : Concatenate  NumInputs=4  Mode=Multidimensional array
  Product : Product  Multiplication=Matrix(*)  OutDataType=sfix(16)  OutScaling=2^0  SaturateOnIntegerOverflow=on  OutDataTypeStr=Inherit: Same as first input
  Reshape{,1..3} (4 alike) : Reshape  OutputDimensionality=Row vector (2-D)
  Sum : Sum  Inputs=+----  OutDataType=sfix(16)  OutScaling=2^0  SaturateOnIntegerOverflow=on
  Sum1 : Sum  Inputs=+---  OutDataType=sfix(16)  OutScaling=2^0  SaturateOnIntegerOverflow=on
  Sum2 : Sum  Inputs=+--  OutDataType=sfix(16)  OutScaling=2^0  SaturateOnIntegerOverflow=on
  Sum3 : Sum  Inputs=+-  OutDataType=sfix(16)  OutScaling=2^0  SaturateOnIntegerOverflow=on
  inv(Polynome Coeff) : Constant  Value="[ -20 10 -2  1/6 ; 70 -34 6.5 -0.5; -84 39 -7 0.5; 35 -15 2.5 -1/6]"  VectorParams1D=off  OutDataType=sfix(16)  OutScaling=2^0  SampleTime=st
  a b c d : Outport
  wires:
  Reshape3/1 -> Matrix Concatenation/4
  Sum3/1 -> Reshape3/1
  Des. Jerk/1 -> Sum3/1
  Des. Acc./1 -> Sum2/1
  Gain2/1 -> Sum3/2, Sum2/2
  Gain1/1 -> Sum2/3, Sum1/3
  Gain/1 -> Sum1/2
  Des. Vel./1 -> Sum1/1
  h/1 -> Sum/5
  g/1 -> Sum1/4, Sum/4
  f/1 -> Gain1/1, Sum/3
  e/1 -> Gain2/1, Gain/1, Sum/2
  Product/1 -> a b c d/1
  inv(Polynome Coeff)/1 -> Product/1
  Reshape2/1 -> Matrix Concatenation/3
  Reshape1/1 -> Matrix Concatenation/2
  Reshape/1 -> Matrix Concatenation/1
  Sum2/1 -> Reshape2/1
  Sum1/1 -> Reshape1/1
  Sum/1 -> Reshape/1
  Des. Pos/1 -> Sum/1
  Matrix Concatenation/1 -> Product/2

== system OneLeg_VR_TouchInput/Trajectory Command/Continous Trajectory Generator/Compute Polynomial Coefficients/Compute tf ==
  pd-p0 : Inport  OutDataType=sfix(16)  OutScaling=2^0
  T : Inport  Port=2  OutDataType=sfix(16)  OutScaling=2^0
  Abs1 : Abs  SaturateOnIntegerOverflow=on
  Abs2 : Abs  SaturateOnIntegerOverflow=on
  Compute T wrt to velocity : Gain  Gain=35./16./maxv  ParameterDataType=sfix(16)  ParameterScaling=2^0  OutDataType=sfix(16)  OutScaling=2^0  SaturateOnIntegerOverflow=on  OutDataTypeStr=Inherit: Same as input  ParamDataTypeStr=Inherit: Same as input
  Compute T  wrt to acceleration : Gain  Gain=84*sqrt(5)./25./max_acc  ParameterDataType=sfix(16)  ParameterScaling=2^0  OutDataType=sfix(16)  OutScaling=2^0  SaturateOnIntegerOverflow=on  OutDataTypeStr=Inherit: Same as input  ParamDataTypeStr=Inherit: Same as input
  Enable Synchronization : Constant  Value=Synchro  OutDataType=sfix(16)  OutScaling=2^0  SampleTime=st
  Math Function1 : Math  Operator=sqrt  SaturateOnIntegerOverflow=on
  MinMax1 : MinMax  Function=max  Inputs=3  SaturateOnIntegerOverflow=on  InputSameDT=on
  MinMax2 : MinMax  Function=max  SaturateOnIntegerOverflow=on  InputSameDT=on
  Reshape1 : Reshape
  Switch : Switch  Threshold=0.5  SaturateOnIntegerOverflow=on
  tf : Outport
  wires:
  Switch/1 -> tf/1
  Enable Synchronization/1 -> Switch/2
  MinMax2/1 -> Switch/1
  Math Function1/1 -> MinMax1/1
  Abs2/1 -> Math Function1/1
  Compute T  wrt to acceleration/1 -> Abs2/1
  pd-p0/1 -> Reshape1/1
  T/1 -> MinMax1/3
  MinMax1/1 -> Switch/3, MinMax2/1
  Abs1/1 -> MinMax1/2
  Compute T wrt to velocity/1 -> Abs1/1  "T"
  Reshape1/1 -> Compute T  wrt to acceleration/1, Compute T wrt to velocity/1

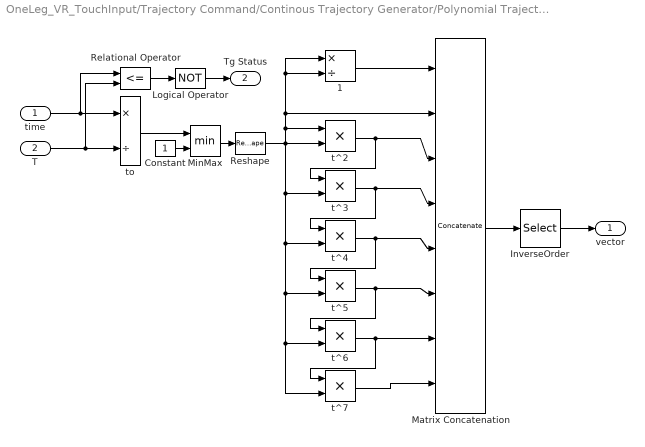
== system OneLeg_VR_TouchInput/Trajectory Command/Continous Trajectory Generator/Polynomial Trajectory/TimeVector ==
  time : Inport  OutDataType=sfix(16)  OutScaling=2^0
  T : Inport  Port=2  OutDataType=sfix(16)  OutScaling=2^0
  1 : Product  Inputs=*/  OutDataType=sfix(16)  OutScaling=2^0  SaturateOnIntegerOverflow=on  InputSameDT=on  OutDataTypeStr=Inherit: Same as first input
  Constant : Constant  OutDataType=sfix(16)  OutScaling=2^0  SampleTime=st
  InverseOrder : Selector  NumberOfDimensions=2  InputPortWidth=3  IndexOptions=Index vector (dialog),Select all  Indices=[ 8 7 6 5 4 3 2 1],-1  OutputSizes=1
  Logical Operator : Logic  Operator=NOT
  Matrix Concatenation : Concatenate  NumInputs=8  Mode=Multidimensional array
  MinMax : MinMax  Inputs=2  SaturateOnIntegerOverflow=on  InputSameDT=on
  Relational Operator : RelationalOperator  Operator=<=  InputSameDT=on
  Reshape : Reshape  OutputDimensionality=Row vector (2-D)
  t^{2..7} (6 alike) : Product  OutDataType=sfix(16)  OutScaling=2^0  SaturateOnIntegerOverflow=on  InputSameDT=on  OutDataTypeStr=Inherit: Same as first input
  to : Product  Inputs=*/  OutDataType=sfix(16)  OutScaling=2^0  SaturateOnIntegerOverflow=on  InputSameDT=on  OutDataTypeStr=Inherit: Same as first input
  vector : Outport
  Tg Status : Outport  Port=2
  wires:
  InverseOrder/1 -> vector/1
  t^7/1 -> Matrix Concatenation/8
  1/1 -> Matrix Concatenation/1
  Reshape/1 -> Matrix Concatenation/2, 1/2, 1/1, t^2/1, t^2/2, t^3/2, t^4/2, t^5/2, t^6/2, t^7/2
  t^2/1 -> Matrix Concatenation/3, t^3/1
  t^3/1 -> Matrix Concatenation/4, t^4/1
  t^4/1 -> Matrix Concatenation/5, t^5/1
  t^5/1 -> Matrix Concatenation/6, t^6/1
  MinMax/1 -> Reshape/1
  t^6/1 -> Matrix Concatenation/7, t^7/1
  Matrix Concatenation/1 -> InverseOrder/1
  Constant/1 -> MinMax/2
  to/1 -> MinMax/1
  time/1 -> to/1, Relational Operator/1
  T/1 -> to/2, Relational Operator/2
  Logical Operator/1 -> Tg Status/1
  Relational Operator/1 -> Logical Operator/1

== system OneLeg_VR_TouchInput/Robot/Leg Tip and Contact Dynamics/Contact Force/Force Law/Contact Force ==
  pos : Inport  OutDataType=sfix(16)  OutScaling=2^0
  vel : Inport  Port=2  OutDataType=sfix(16)  OutScaling=2^0
  Action Port : ActionPort  InitializeStates=reset  ActionType=then
  Constant : Constant  Value=0  OutDataType=sfix(16)  OutScaling=2^0
  Damping : Gain  Gain=ground.damping  Multiplication=Matrix(K*u)  ParameterDataType=sfix(16)  ParameterScaling=2^0  OutDataType=sfix(16)  OutScaling=2^0  SaturateOnIntegerOverflow=on  OutDataTypeStr=Inherit: Same as input  ParamDataTypeStr=Inherit: Same as input
  Memory : Memory  X0=1
  Saturation : Saturate  UpperLimit=[inf inf inf]  LowerLimit=[-inf 0 -inf]
  Spring : Gain  Gain=-ground.stiffness  ParameterDataType=sfix(16)  ParameterScaling=2^0  OutDataType=sfix(16)  OutScaling=2^0  SaturateOnIntegerOverflow=on  OutDataTypeStr=Inherit: Same as input  ParamDataTypeStr=Inherit: Same as input
  Store Initial Value : Subsystem  TreatAsAtomicUnit=on
  Sum : Sum  Inputs=--  OutDataType=sfix(16)  OutScaling=2^0  SaturateOnIntegerOverflow=on
  Sum1 : Sum  Inputs=+-  OutDataType=sfix(16)  OutScaling=2^0  SaturateOnIntegerOverflow=on
  force : Outport  OutDataType=sfix(16)  OutScaling=2^0  InitialOutput=0
  wires:
  Memory/1 -> Store Initial Value/Enable
  Store Initial Value/1(Out1) -> Sum1/1
  Sum/1 -> Saturation/1
  Sum1/1 -> Spring/1
  Spring/1 -> Sum/1
  Damping/1 -> Sum/2
  Constant/1 -> Memory/1
  vel/1 -> Damping/1
  pos/1 -> Store Initial Value/1(In1), Sum1/2
  Saturation/1 -> force/1

== system OneLeg_VR_TouchInput/Robot/Leg Tip and Contact Dynamics/Contact Force/Force Law/Zero Force ==
  Action Port : ActionPort  ActionType=else
  Zero Force : Constant  Value=[0;0;0]  OutDataType=sfix(16)  OutScaling=2^0
  force : Outport  OutDataType=sfix(16)  OutScaling=2^0  InitialOutput=0
  wires:
  Zero Force/1 -> force/1

== system OneLeg_VR_TouchInput/Robot/Leg Tip and Contact Dynamics/Contact Force/Force Law/Contact Force/Store Initial Value ==
  In1 : Inport  OutDataType=sfix(16)  OutScaling=2^0
  Enable : EnablePort
  Set Y=0 : Gain  Gain=[1 0 1]  ParameterDataType=sfix(16)  ParameterScaling=2^0  OutDataType=sfix(16)  OutScaling=2^0  SaturateOnIntegerOverflow=on  OutDataTypeStr=Inherit: Same as input  ParamDataTypeStr=Inherit: Same as input
  Out1 : Outport  OutDataType=sfix(16)  OutScaling=2^0
  wires:
  Set Y=0/1 -> Out1/1
  In1/1 -> Set Y=0/1
